simulink library "wheels"  (R2022b)
settings: Solver=VariableStepAuto  StartTime=0.0  StopTime=10.0  RelTol=1e-3
undefined symbols (not defined in the file): raptor_xcp_function
libraries: Raptor_lib x44
settings Model: Creator=serga  LastModifiedBy=serga

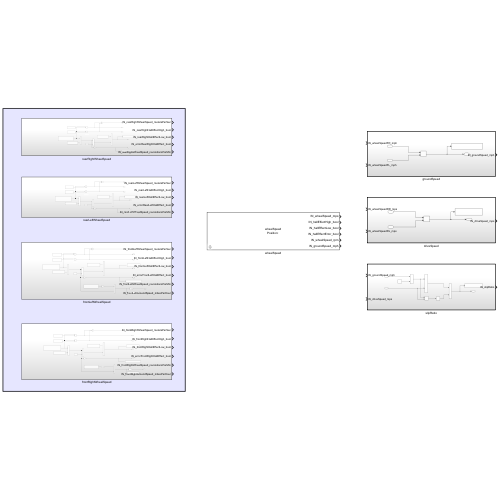
[thumbnail: Simulink's stored preview of the top-level diagram]
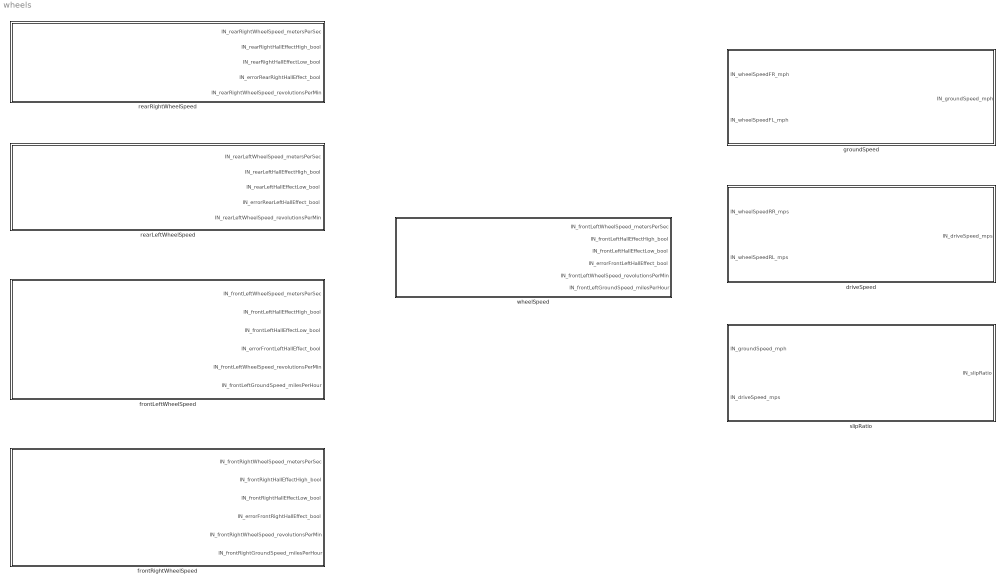
== system wheels ==
  driveSpeed : Subsystem  TreatAsAtomicUnit=on
  frontLeftWheelSpeed : Subsystem
  frontRightWheelSpeed : Subsystem
  groundSpeed : Subsystem  TreatAsAtomicUnit=on
  rearLeftWheelSpeed : Subsystem
  rearRightWheelSpeed : Subsystem
  slipRatio : Subsystem  TreatAsAtomicUnit=on
  wheelSpeed : Subsystem  mask{pos=''}
      mask prompts: pos "Position"
      mask Display:
      | disp(['wheelSpeed\n' ...
      |     'Position: ' pos]);
      | port_label('output', 1, ['IN_wheelSpeed' pos '_mps']);
      | port_label('output', 2, ['IN_hallEffectHigh' pos '_bool']);
      | port_label('output', 3, ['IN_hallEffectLow' pos '_bool']);
      | port_label('output', 4, ['IN_hallEffectError' pos '_bool']);
      | port_label('output', 5, ['IN_wheelSpeed' pos '_rpm']);
      | port_label('output', 6, ['IN_groundSpeed' pos '_mph']);

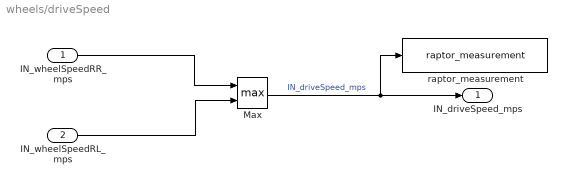
== system wheels/driveSpeed ==
  IN_wheelSpeedRR_mps : Inport
  IN_wheelSpeedRL_mps : Inport  Port=2
  Max : MinMax  Function=max  Inputs=2
  raptor_measurement : Raptor_lib/Data Storage/raptor_measurement  paramName='DataName'  nameSource=Input Wire  calDispType=Number  calEnum={'False', 'True'}  calGain=1.0  calOffset=0.0  calMax=inf  calMin=-inf  calFormat='-1'  calUnit=''  calHelp=''  calAccess=1  calFunction=raptor_xcp_function(gcb)  calVisible=on
      settings: SourceProductName=Raptor
  IN_driveSpeed_mps : Outport
  wires:
  IN_wheelSpeedRL_mps/1 -> Max/2
  Max/1 -> raptor_measurement/1, IN_driveSpeed_mps/1  "IN_driveSpeed_mps"
  IN_wheelSpeedRR_mps/1 -> Max/1

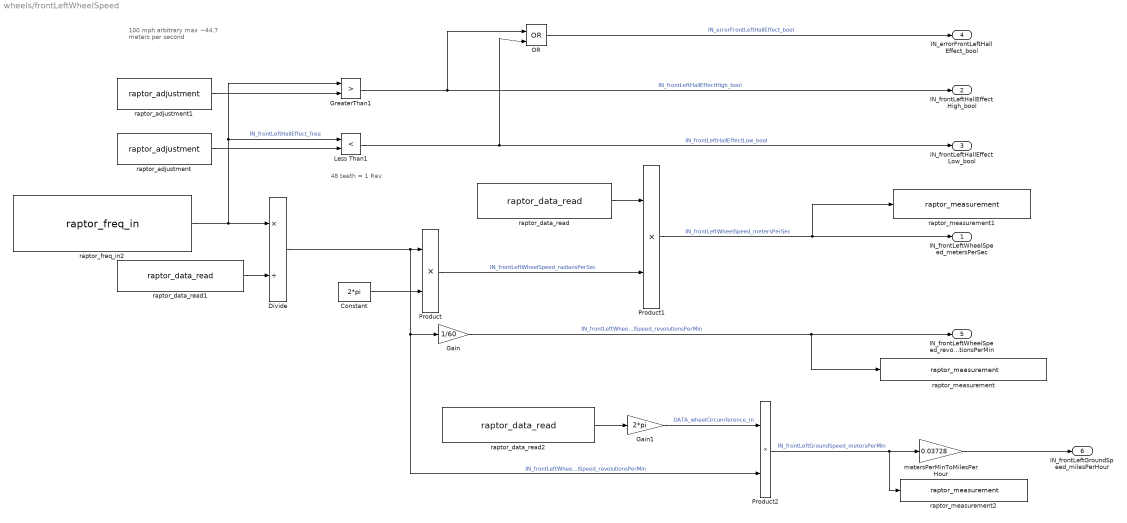
== system wheels/frontLeftWheelSpeed ==
  note: 48 teeth = 1 Rev
  note: 100 mph arbitrary max
      | ~44.7 meters per second
  Constant : Constant  Value=2*pi
  Divide : Product  Inputs=*/
  Gain : Gain  Gain=1/60
  Gain1 : Gain  Gain=2*pi
  GreaterThan1 : RelationalOperator  Operator=>  OutDataTypeStr=boolean  RndMeth=Simplest  InputSameDT=off
  Less Than1 : RelationalOperator  Operator=<  OutDataTypeStr=boolean  RndMeth=Simplest  InputSameDT=off
  OR : Logic  Operator=OR  IconShape=distinctive  AllPortsSameDT=off  OutDataTypeStr=boolean
  Product : Product
  Product1 : Product
  Product2 : Product
  metersPerMinToMilesPerHour : Gain  Gain=0.03728
  raptor_adjustment : Raptor_lib/Data Storage/raptor_adjustment  paramName='IN_frontLeftHallEffectLow_freq'  nameSource=Parameter  initValue=0  dataType=single  storage=Calibration  calDispType=Number  calEnum={'False', 'True'}  calGain=1.0  calOffset=0.0  calMax=inf  calMin=-inf  calFormat='-1'  calUnit=''  calHelp=''  calAccess=1  calFunction=raptor_xcp_function(gcb)  calDispHeaders=off  calColHeaders={'Col1' 'Col2' 'Col3'}  calRowHeaders={'Row1' 'Row2' 'Row3'}
      settings: SourceProductName=Raptor
  raptor_adjustment1 : Raptor_lib/Data Storage/raptor_adjustment  paramName='IN_frontLeftHallEffectHigh_freq'  nameSource=Parameter  initValue=1680  dataType=single  storage=Calibration  calDispType=Number  calEnum={'False', 'True'}  calGain=1.0  calOffset=0.0  calMax=inf  calMin=-inf  calFormat='-1'  calUnit=''  calHelp=''  calAccess=1  calFunction=raptor_xcp_function(gcb)  calDispHeaders=off  calColHeaders={'Col1' 'Col2' 'Col3'}  calRowHeaders={'Row1' 'Row2' 'Row3'}
      settings: SourceProductName=Raptor
  raptor_data_read : Raptor_lib/Data Storage/raptor_data_read  dataName='DATA_unloadedWheelRadius_m'  dataShape=Scalar  idxSource=Input  idxRow=1  idxCol=1
      settings: SourceProductName=Raptor
  raptor_data_read1 : Raptor_lib/Data Storage/raptor_data_read  dataName='DATA_wheelTooth_ct'  dataShape=Scalar  idxSource=Input  idxRow=1  idxCol=1
      settings: SourceProductName=Raptor
  raptor_data_read2 : Raptor_lib/Data Storage/raptor_data_read  dataName='DATA_unloadedWheelRadius_m'  dataShape=Scalar  idxSource=Input  idxRow=1  idxCol=1
      settings: SourceProductName=Raptor
  raptor_freq_in2 : Raptor_lib/Input & Output/raptor_freq_in  resourceValues=INPUT41|INPUT42|INPUT43|INPUT44|INPUT45|(None)  resource=INPUT43  pullUDValues=[]  pullUD=[]  interfaceValues=[]  interface=[]  hasDuty=off  hasEdgeCount='RAPTOR MASK DEFAULT'
      settings: SourceProductName=Raptor
  raptor_measurement : Raptor_lib/Data Storage/raptor_measurement  paramName='DataName'  nameSource=Input Wire  calDispType=Number  calEnum={'False', 'True'}  calGain=1.0  calOffset=0.0  calMax=inf  calMin=-inf  calFormat='-1'  calUnit=''  calHelp=''  calAccess=1  calFunction=raptor_xcp_function(gcb)  calVisible=on
      settings: SourceProductName=Raptor
  raptor_measurement1 : Raptor_lib/Data Storage/raptor_measurement  paramName='DataName'  nameSource=Input Wire  calDispType=Number  calEnum={'False', 'True'}  calGain=1.0  calOffset=0.0  calMax=inf  calMin=-inf  calFormat='-1'  calUnit=''  calHelp=''  calAccess=1  calFunction=raptor_xcp_function(gcb)  calVisible=on
      settings: SourceProductName=Raptor
  raptor_measurement2 : Raptor_lib/Data Storage/raptor_measurement  paramName='DataName'  nameSource=Input Wire  calDispType=Number  calEnum={'False', 'True'}  calGain=1.0  calOffset=0.0  calMax=inf  calMin=-inf  calFormat='-1'  calUnit=''  calHelp=''  calAccess=1  calFunction=raptor_xcp_function(gcb)  calVisible=on
      settings: SourceProductName=Raptor
  IN_frontLeftWheelSpeed_metersPerSec : Outport
  IN_frontLeftHallEffectHigh_bool : Outport  Port=2
  IN_frontLeftHallEffectLow_bool : Outport  Port=3
  IN_errorFrontLeftHallEffect_bool : Outport  Port=4
  IN_frontLeftWheelSpeed_revolutionsPerMin : Outport  Port=5
  IN_frontLeftGroundSpeed_milesPerHour : Outport  Port=6
  wires:
  Product2/1 -> raptor_measurement2/1, metersPerMinToMilesPerHour/1  "IN_frontLeftGroundSpeed_metersPerMin"
  Divide/1 -> Product2/2, Gain/1, Product/1  "IN_frontLeftWheelSpeed_revolutionsPerMin"
  Gain1/1 -> Product2/1  "DATA_wheelCircumference_m"
  raptor_data_read/1 -> Product1/1
  raptor_data_read2/1 -> Gain1/1
  Less Than1/1 -> IN_frontLeftHallEffectLow_bool/1, OR/2  "IN_frontLeftHallEffectLow_bool"
  raptor_freq_in2/1 -> Less Than1/1, GreaterThan1/1, Divide/1  "IN_frontLeftHallEffect_freq"
  metersPerMinToMilesPerHour/1 -> IN_frontLeftGroundSpeed_milesPerHour/1
  Constant/1 -> Product/2
  raptor_adjustment/1 -> Less Than1/2
  OR/1 -> IN_errorFrontLeftHallEffect_bool/1  "IN_errorFrontLeftHallEffect_bool"
  raptor_adjustment1/1 -> GreaterThan1/2
  raptor_data_read1/1 -> Divide/2
  Product1/1 -> raptor_measurement1/1, IN_frontLeftWheelSpeed_metersPerSec/1  "IN_frontLeftWheelSpeed_metersPerSec"
  Gain/1 -> raptor_measurement/1, IN_frontLeftWheelSpeed_revolutionsPerMin/1  "IN_frontLeftWheelSpeed_revolutionsPerMin"
  Product/1 -> Product1/2  "IN_frontLeftWheelSpeed_radiansPerSec"
  GreaterThan1/1 -> IN_frontLeftHallEffectHigh_bool/1, OR/1  "IN_frontLeftHallEffectHigh_bool"

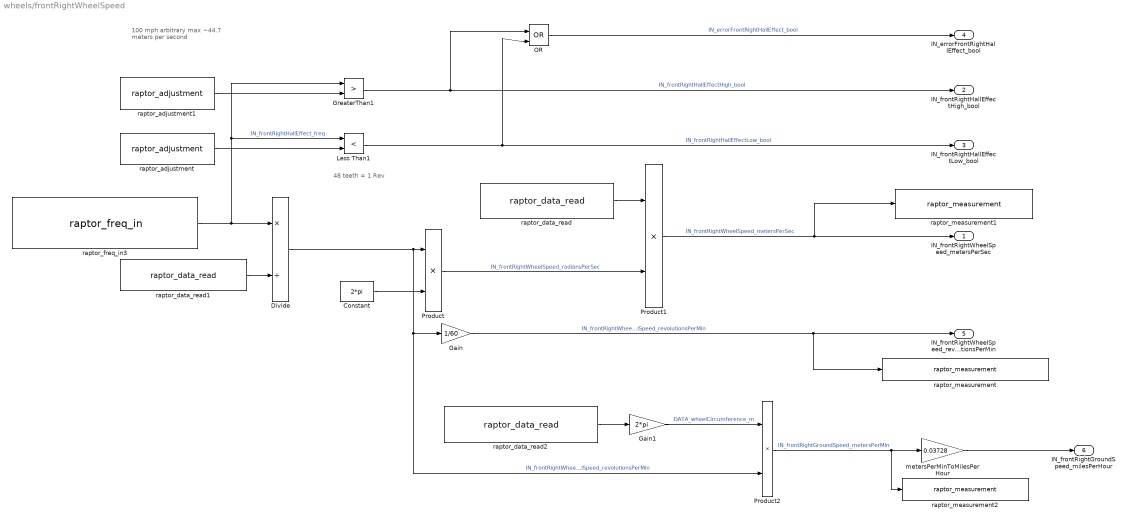
== system wheels/frontRightWheelSpeed ==
  note: 100 mph arbitrary max
      | ~44.7 meters per second
  note: 48 teeth = 1 Rev
  Constant : Constant  Value=2*pi
  Divide : Product  Inputs=*/
  Gain : Gain  Gain=1/60
  Gain1 : Gain  Gain=2*pi
  GreaterThan1 : RelationalOperator  Operator=>  OutDataTypeStr=boolean  RndMeth=Simplest  InputSameDT=off
  Less Than1 : RelationalOperator  Operator=<  OutDataTypeStr=boolean  RndMeth=Simplest  InputSameDT=off
  OR : Logic  Operator=OR  IconShape=distinctive  AllPortsSameDT=off  OutDataTypeStr=boolean
  Product : Product
  Product1 : Product
  Product2 : Product
  metersPerMinToMilesPerHour : Gain  Gain=0.03728
  raptor_adjustment : Raptor_lib/Data Storage/raptor_adjustment  paramName='IN_frontRightHallEffectLow_freq'  nameSource=Parameter  initValue=0  dataType=single  storage=Calibration  calDispType=Number  calEnum={'False', 'True'}  calGain=1.0  calOffset=0.0  calMax=inf  calMin=-inf  calFormat='-1'  calUnit=''  calHelp=''  calAccess=1  calFunction=raptor_xcp_function(gcb)  calDispHeaders=off  calColHeaders={'Col1' 'Col2' 'Col3'}  calRowHeaders={'Row1' 'Row2' 'Row3'}
      settings: SourceProductName=Raptor
  raptor_adjustment1 : Raptor_lib/Data Storage/raptor_adjustment  paramName='IN_frontRightHallEffectHigh_freq'  nameSource=Parameter  initValue=1680  dataType=single  storage=Calibration  calDispType=Number  calEnum={'False', 'True'}  calGain=1.0  calOffset=0.0  calMax=inf  calMin=-inf  calFormat='-1'  calUnit=''  calHelp=''  calAccess=1  calFunction=raptor_xcp_function(gcb)  calDispHeaders=off  calColHeaders={'Col1' 'Col2' 'Col3'}  calRowHeaders={'Row1' 'Row2' 'Row3'}
      settings: SourceProductName=Raptor
  raptor_data_read : Raptor_lib/Data Storage/raptor_data_read  dataName='DATA_unloadedWheelRadius_m'  dataShape=Scalar  idxSource=Input  idxRow=1  idxCol=1
      settings: SourceProductName=Raptor
  raptor_data_read1 : Raptor_lib/Data Storage/raptor_data_read  dataName='DATA_wheelTooth_ct'  dataShape=Scalar  idxSource=Input  idxRow=1  idxCol=1
      settings: SourceProductName=Raptor
  raptor_data_read2 : Raptor_lib/Data Storage/raptor_data_read  dataName='DATA_unloadedWheelRadius_m'  dataShape=Scalar  idxSource=Input  idxRow=1  idxCol=1
      settings: SourceProductName=Raptor
  raptor_freq_in3 : Raptor_lib/Input & Output/raptor_freq_in  resourceValues=INPUT41|INPUT42|INPUT43|INPUT44|INPUT45|(None)  resource=INPUT44  pullUDValues=[]  pullUD=[]  interfaceValues=[]  interface=[]  hasDuty=off  hasEdgeCount='RAPTOR MASK DEFAULT'
      settings: SourceProductName=Raptor
  raptor_measurement : Raptor_lib/Data Storage/raptor_measurement  paramName='DataName'  nameSource=Input Wire  calDispType=Number  calEnum={'False', 'True'}  calGain=1.0  calOffset=0.0  calMax=inf  calMin=-inf  calFormat='-1'  calUnit=''  calHelp=''  calAccess=1  calFunction=raptor_xcp_function(gcb)  calVisible=on
      settings: SourceProductName=Raptor
  raptor_measurement1 : Raptor_lib/Data Storage/raptor_measurement  paramName='DataName'  nameSource=Input Wire  calDispType=Number  calEnum={'False', 'True'}  calGain=1.0  calOffset=0.0  calMax=inf  calMin=-inf  calFormat='-1'  calUnit=''  calHelp=''  calAccess=1  calFunction=raptor_xcp_function(gcb)  calVisible=on
      settings: SourceProductName=Raptor
  raptor_measurement2 : Raptor_lib/Data Storage/raptor_measurement  paramName='DataName'  nameSource=Input Wire  calDispType=Number  calEnum={'False', 'True'}  calGain=1.0  calOffset=0.0  calMax=inf  calMin=-inf  calFormat='-1'  calUnit=''  calHelp=''  calAccess=1  calFunction=raptor_xcp_function(gcb)  calVisible=on
      settings: SourceProductName=Raptor
  IN_frontRightWheelSpeed_metersPerSec : Outport
  IN_frontRightHallEffectHigh_bool : Outport  Port=2
  IN_frontRightHallEffectLow_bool : Outport  Port=3
  IN_errorFrontRightHallEffect_bool : Outport  Port=4
  IN_frontRightWheelSpeed_revolutionsPerMin : Outport  Port=5
  IN_frontRightGroundSpeed_milesPerHour : Outport  Port=6
  wires:
  raptor_adjustment/1 -> Less Than1/2
  raptor_freq_in3/1 -> Less Than1/1, GreaterThan1/1, Divide/1  "IN_frontRightHallEffect_freq"
  raptor_adjustment1/1 -> GreaterThan1/2
  OR/1 -> IN_errorFrontRightHallEffect_bool/1  "IN_errorFrontRightHallEffect_bool"
  GreaterThan1/1 -> IN_frontRightHallEffectHigh_bool/1, OR/1  "IN_frontRightHallEffectHigh_bool"
  Less Than1/1 -> IN_frontRightHallEffectLow_bool/1, OR/2  "IN_frontRightHallEffectLow_bool"
  Gain/1 -> raptor_measurement/1, IN_frontRightWheelSpeed_revolutionsPerMin/1  "IN_frontRightWheelSpeed_revolutionsPerMin"
  raptor_data_read1/1 -> Divide/2
  raptor_data_read/1 -> Product1/1
  Constant/1 -> Product/2
  Product1/1 -> raptor_measurement1/1, IN_frontRightWheelSpeed_metersPerSec/1  "IN_frontRightWheelSpeed_metersPerSec"
  Product/1 -> Product1/2  "IN_frontRightWheelSpeed_radiansPerSec"
  Product2/1 -> raptor_measurement2/1, metersPerMinToMilesPerHour/1  "IN_frontRightGroundSpeed_metersPerMin"
  Gain1/1 -> Product2/1  "DATA_wheelCircumference_m"
  Divide/1 -> Product2/2, Gain/1, Product/1  "IN_frontRightWheelSpeed_revolutionsPerMin"
  raptor_data_read2/1 -> Gain1/1
  metersPerMinToMilesPerHour/1 -> IN_frontRightGroundSpeed_milesPerHour/1

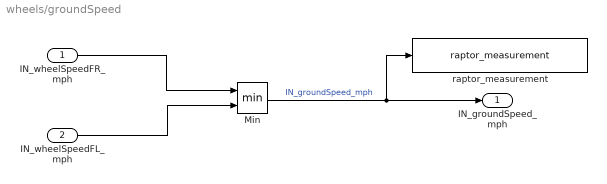
== system wheels/groundSpeed ==
  IN_wheelSpeedFR_mph : Inport
  IN_wheelSpeedFL_mph : Inport  Port=2
  Min : MinMax  Inputs=2
  raptor_measurement : Raptor_lib/Data Storage/raptor_measurement  paramName='DataName'  nameSource=Input Wire  calDispType=Number  calEnum={'False', 'True'}  calGain=1.0  calOffset=0.0  calMax=inf  calMin=-inf  calFormat='-1'  calUnit=''  calHelp=''  calAccess=1  calFunction=raptor_xcp_function(gcb)  calVisible=on
      settings: SourceProductName=Raptor
  IN_groundSpeed_mph : Outport
  wires:
  IN_wheelSpeedFR_mph/1 -> Min/1
  IN_wheelSpeedFL_mph/1 -> Min/2
  Min/1 -> raptor_measurement/1, IN_groundSpeed_mph/1  "IN_groundSpeed_mph"

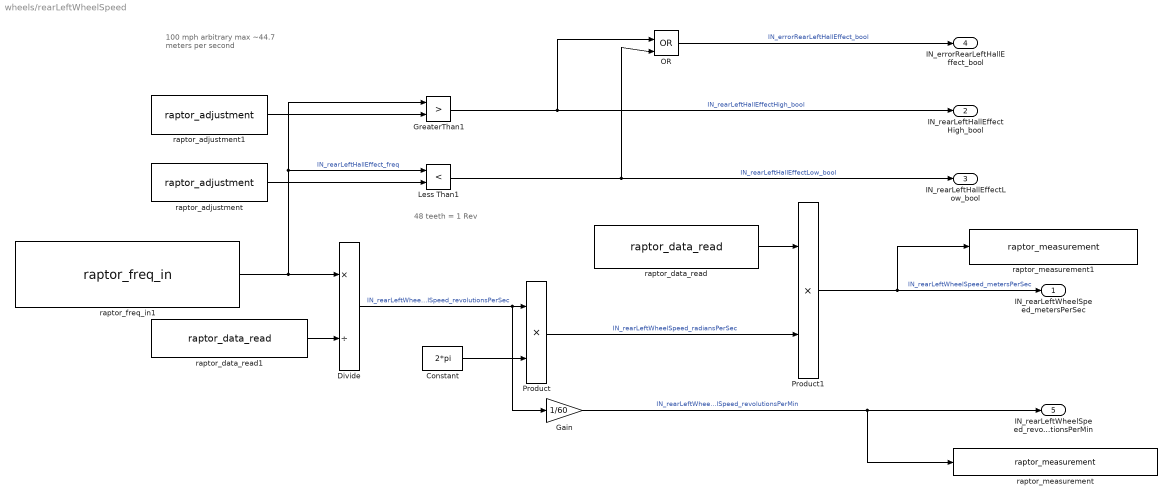
== system wheels/rearLeftWheelSpeed ==
  note: 100 mph arbitrary max
      | ~44.7 meters per second
  note: 48 teeth = 1 Rev
  Constant : Constant  Value=2*pi
  Divide : Product  Inputs=*/
  Gain : Gain  Gain=1/60
  GreaterThan1 : RelationalOperator  Operator=>  OutDataTypeStr=boolean  RndMeth=Simplest  InputSameDT=off
  Less Than1 : RelationalOperator  Operator=<  OutDataTypeStr=boolean  RndMeth=Simplest  InputSameDT=off
  OR : Logic  Operator=OR  IconShape=distinctive  AllPortsSameDT=off  OutDataTypeStr=boolean
  Product : Product
  Product1 : Product
  raptor_adjustment : Raptor_lib/Data Storage/raptor_adjustment  paramName='IN_rearLeftHallEffectLow_freq'  nameSource=Parameter  initValue=0  dataType=single  storage=Calibration  calDispType=Number  calEnum={'False', 'True'}  calGain=1.0  calOffset=0.0  calMax=inf  calMin=-inf  calFormat='-1'  calUnit=''  calHelp=''  calAccess=1  calFunction=raptor_xcp_function(gcb)  calDispHeaders=off  calColHeaders={'Col1' 'Col2' 'Col3'}  calRowHeaders={'Row1' 'Row2' 'Row3'}
      settings: SourceProductName=Raptor
  raptor_adjustment1 : Raptor_lib/Data Storage/raptor_adjustment  paramName='IN_rearLeftHallEffectHigh_freq'  nameSource=Parameter  initValue=1680  dataType=single  storage=Calibration  calDispType=Number  calEnum={'False', 'True'}  calGain=1.0  calOffset=0.0  calMax=inf  calMin=-inf  calFormat='-1'  calUnit=''  calHelp=''  calAccess=1  calFunction=raptor_xcp_function(gcb)  calDispHeaders=off  calColHeaders={'Col1' 'Col2' 'Col3'}  calRowHeaders={'Row1' 'Row2' 'Row3'}
      settings: SourceProductName=Raptor
  raptor_data_read : Raptor_lib/Data Storage/raptor_data_read  dataName='DATA_unloadedWheelRadius_m'  dataShape=Scalar  idxSource=Input  idxRow=1  idxCol=1
      settings: SourceProductName=Raptor
  raptor_data_read1 : Raptor_lib/Data Storage/raptor_data_read  dataName='DATA_wheelTooth_ct'  dataShape=Scalar  idxSource=Input  idxRow=1  idxCol=1
      settings: SourceProductName=Raptor
  raptor_freq_in1 : Raptor_lib/Input & Output/raptor_freq_in  resourceValues=INPUT41|INPUT42|INPUT43|INPUT44|INPUT45|(None)  resource=INPUT42  pullUDValues=[]  pullUD=[]  interfaceValues=[]  interface=[]  hasDuty=off  hasEdgeCount='RAPTOR MASK DEFAULT'
      settings: SourceProductName=Raptor
  raptor_measurement : Raptor_lib/Data Storage/raptor_measurement  paramName='DataName'  nameSource=Input Wire  calDispType=Number  calEnum={'False', 'True'}  calGain=1.0  calOffset=0.0  calMax=inf  calMin=-inf  calFormat='-1'  calUnit=''  calHelp=''  calAccess=1  calFunction=raptor_xcp_function(gcb)  calVisible=on
      settings: SourceProductName=Raptor
  raptor_measurement1 : Raptor_lib/Data Storage/raptor_measurement  paramName='DataName'  nameSource=Input Wire  calDispType=Number  calEnum={'False', 'True'}  calGain=1.0  calOffset=0.0  calMax=inf  calMin=-inf  calFormat='-1'  calUnit=''  calHelp=''  calAccess=1  calFunction=raptor_xcp_function(gcb)  calVisible=on
      settings: SourceProductName=Raptor
  IN_rearLeftWheelSpeed_metersPerSec : Outport
  IN_rearLeftHallEffectHigh_bool : Outport  Port=2
  IN_rearLeftHallEffectLow_bool : Outport  Port=3
  IN_errorRearLeftHallEffect_bool : Outport  Port=4
  IN_rearLeftWheelSpeed_revolutionsPerMin : Outport  Port=5
  wires:
  raptor_adjustment/1 -> Less Than1/2
  raptor_freq_in1/1 -> Less Than1/1, GreaterThan1/1, Divide/1  "IN_rearLeftHallEffect_freq"
  raptor_adjustment1/1 -> GreaterThan1/2
  OR/1 -> IN_errorRearLeftHallEffect_bool/1  "IN_errorRearLeftHallEffect_bool"
  GreaterThan1/1 -> IN_rearLeftHallEffectHigh_bool/1, OR/1  "IN_rearLeftHallEffectHigh_bool"
  Less Than1/1 -> IN_rearLeftHallEffectLow_bool/1, OR/2  "IN_rearLeftHallEffectLow_bool"
  Gain/1 -> IN_rearLeftWheelSpeed_revolutionsPerMin/1, raptor_measurement/1  "IN_rearLeftWheelSpeed_revolutionsPerMin"
  raptor_data_read1/1 -> Divide/2
  raptor_data_read/1 -> Product1/1
  Divide/1 -> Gain/1, Product/1  "IN_rearLeftWheelSpeed_revolutionsPerSec"
  Constant/1 -> Product/2
  Product1/1 -> raptor_measurement1/1, IN_rearLeftWheelSpeed_metersPerSec/1  "IN_rearLeftWheelSpeed_metersPerSec"
  Product/1 -> Product1/2  "IN_rearLeftWheelSpeed_radiansPerSec"

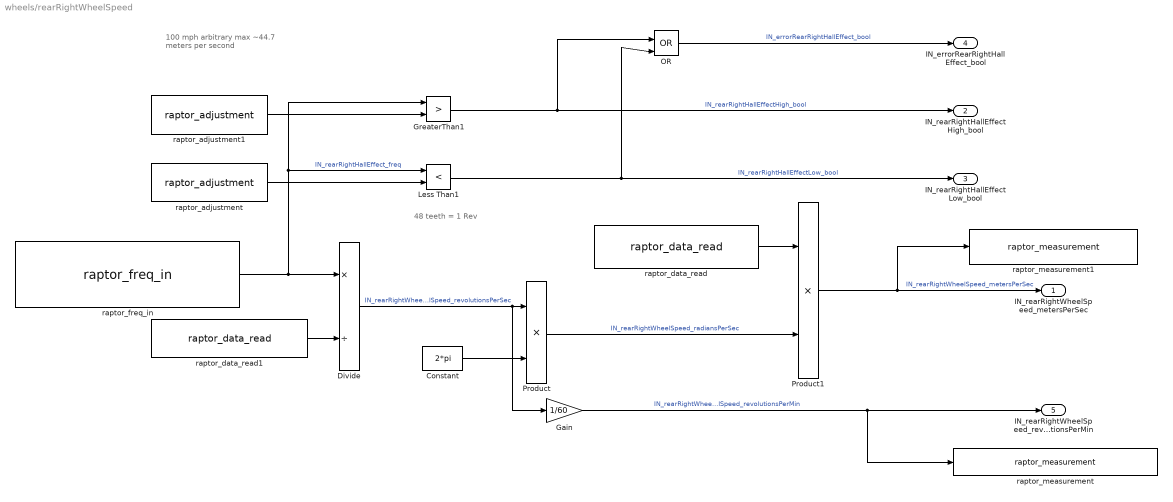
== system wheels/rearRightWheelSpeed ==
  note: 100 mph arbitrary max
      | ~44.7 meters per second
  note: 48 teeth = 1 Rev
  Constant : Constant  Value=2*pi
  Divide : Product  Inputs=*/
  Gain : Gain  Gain=1/60
  GreaterThan1 : RelationalOperator  Operator=>  OutDataTypeStr=boolean  RndMeth=Simplest  InputSameDT=off
  Less Than1 : RelationalOperator  Operator=<  OutDataTypeStr=boolean  RndMeth=Simplest  InputSameDT=off
  OR : Logic  Operator=OR  IconShape=distinctive  AllPortsSameDT=off  OutDataTypeStr=boolean
  Product : Product
  Product1 : Product
  raptor_adjustment : Raptor_lib/Data Storage/raptor_adjustment  paramName='IN_rearRightHallEffectLow_freq'  nameSource=Parameter  initValue=0  dataType=single  storage=Calibration  calDispType=Number  calEnum={'False', 'True'}  calGain=1.0  calOffset=0.0  calMax=inf  calMin=-inf  calFormat='-1'  calUnit=''  calHelp=''  calAccess=1  calFunction=raptor_xcp_function(gcb)  calDispHeaders=off  calColHeaders={'Col1' 'Col2' 'Col3'}  calRowHeaders={'Row1' 'Row2' 'Row3'}
      settings: SourceProductName=Raptor
  raptor_adjustment1 : Raptor_lib/Data Storage/raptor_adjustment  paramName='IN_rearRightHallEffectHigh_freq'  nameSource=Parameter  initValue=1680  dataType=single  storage=Calibration  calDispType=Number  calEnum={'False', 'True'}  calGain=1.0  calOffset=0.0  calMax=inf  calMin=-inf  calFormat='-1'  calUnit=''  calHelp=''  calAccess=1  calFunction=raptor_xcp_function(gcb)  calDispHeaders=off  calColHeaders={'Col1' 'Col2' 'Col3'}  calRowHeaders={'Row1' 'Row2' 'Row3'}
      settings: SourceProductName=Raptor
  raptor_data_read : Raptor_lib/Data Storage/raptor_data_read  dataName='DATA_unloadedWheelRadius_m'  dataShape=Scalar  idxSource=Input  idxRow=1  idxCol=1
      settings: SourceProductName=Raptor
  raptor_data_read1 : Raptor_lib/Data Storage/raptor_data_read  dataName='DATA_wheelTooth_ct'  dataShape=Scalar  idxSource=Input  idxRow=1  idxCol=1
      settings: SourceProductName=Raptor
  raptor_freq_in : Raptor_lib/Input & Output/raptor_freq_in  resourceValues=INPUT41|INPUT42|INPUT43|INPUT44|INPUT45|(None)  resource=INPUT41  pullUDValues=[]  pullUD=[]  interfaceValues=[]  interface=[]  hasDuty=off  hasEdgeCount='RAPTOR MASK DEFAULT'
      settings: SourceProductName=Raptor
  raptor_measurement : Raptor_lib/Data Storage/raptor_measurement  paramName='DataName'  nameSource=Input Wire  calDispType=Number  calEnum={'False', 'True'}  calGain=1.0  calOffset=0.0  calMax=inf  calMin=-inf  calFormat='-1'  calUnit=''  calHelp=''  calAccess=1  calFunction=raptor_xcp_function(gcb)  calVisible=on
      settings: SourceProductName=Raptor
  raptor_measurement1 : Raptor_lib/Data Storage/raptor_measurement  paramName='DataName'  nameSource=Input Wire  calDispType=Number  calEnum={'False', 'True'}  calGain=1.0  calOffset=0.0  calMax=inf  calMin=-inf  calFormat='-1'  calUnit=''  calHelp=''  calAccess=1  calFunction=raptor_xcp_function(gcb)  calVisible=on
      settings: SourceProductName=Raptor
  IN_rearRightWheelSpeed_metersPerSec : Outport
  IN_rearRightHallEffectHigh_bool : Outport  Port=2
  IN_rearRightHallEffectLow_bool : Outport  Port=3
  IN_errorRearRightHallEffect_bool : Outport  Port=4
  IN_rearRightWheelSpeed_revolutionsPerMin : Outport  Port=5
  wires:
  raptor_data_read1/1 -> Divide/2
  Divide/1 -> Gain/1, Product/1  "IN_rearRightWheelSpeed_revolutionsPerSec"
  Constant/1 -> Product/2
  Product/1 -> Product1/2  "IN_rearRightWheelSpeed_radiansPerSec"
  raptor_data_read/1 -> Product1/1
  Product1/1 -> raptor_measurement1/1, IN_rearRightWheelSpeed_metersPerSec/1  "IN_rearRightWheelSpeed_metersPerSec"
  raptor_freq_in/1 -> Less Than1/1, GreaterThan1/1, Divide/1  "IN_rearRightHallEffect_freq"
  raptor_adjustment1/1 -> GreaterThan1/2
  raptor_adjustment/1 -> Less Than1/2
  Less Than1/1 -> IN_rearRightHallEffectLow_bool/1, OR/2  "IN_rearRightHallEffectLow_bool"
  OR/1 -> IN_errorRearRightHallEffect_bool/1  "IN_errorRearRightHallEffect_bool"
  GreaterThan1/1 -> IN_rearRightHallEffectHigh_bool/1, OR/1  "IN_rearRightHallEffectHigh_bool"
  Gain/1 -> IN_rearRightWheelSpeed_revolutionsPerMin/1, raptor_measurement/1  "IN_rearRightWheelSpeed_revolutionsPerMin"

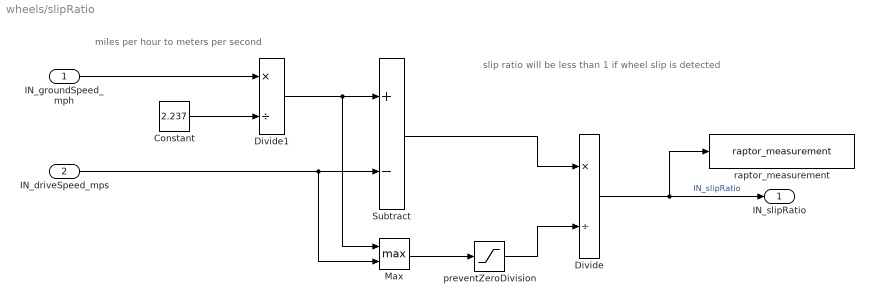
== system wheels/slipRatio ==
  note: slip ratio will be less than 1 if wheel slip is detected
  note: miles per hour to meters per second
  IN_groundSpeed_mph : Inport
  IN_driveSpeed_mps : Inport  Port=2
  Constant : Constant  Value=2.237
  Divide : Product  Inputs=*/
  Divide1 : Product  Inputs=*/
  Max : MinMax  Function=max  Inputs=2
  Subtract : Sum  Inputs=+-
  preventZeroDivision : Saturate  UpperLimit=1000  LowerLimit=0.0001
  raptor_measurement : Raptor_lib/Data Storage/raptor_measurement  paramName='DataName'  nameSource=Input Wire  calDispType=Number  calEnum={'False', 'True'}  calGain=1.0  calOffset=0.0  calMax=inf  calMin=-inf  calFormat='-1'  calUnit=''  calHelp=''  calAccess=1  calFunction=raptor_xcp_function(gcb)  calVisible=on
      settings: SourceProductName=Raptor
  IN_slipRatio : Outport
  wires:
  Divide/1 -> raptor_measurement/1, IN_slipRatio/1  "IN_slipRatio"
  IN_groundSpeed_mph/1 -> Divide1/1
  Constant/1 -> Divide1/2
  IN_driveSpeed_mps/1 -> Max/2, Subtract/2
  Divide1/1 -> Max/1, Subtract/1
  Subtract/1 -> Divide/1
  Max/1 -> preventZeroDivision/1
  preventZeroDivision/1 -> Divide/2

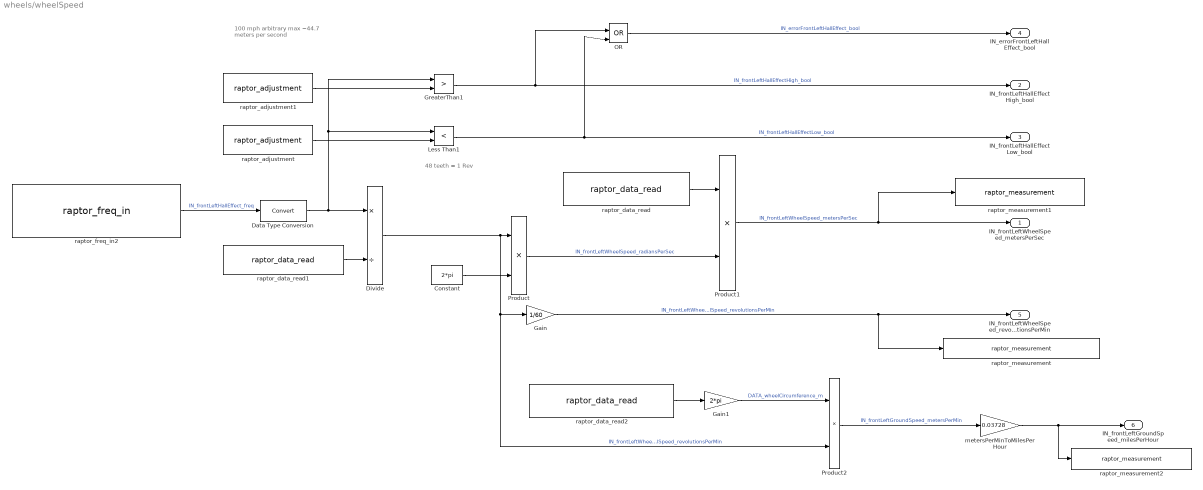
== system wheels/wheelSpeed ==
  note: 48 teeth = 1 Rev
  note: 100 mph arbitrary max
      | ~44.7 meters per second
  Constant : Constant  Value=2*pi
  Data Type Conversion : DataTypeConversion  SaturateOnIntegerOverflow=off  RndMeth=Floor
  Divide : Product  Inputs=*/
  Gain : Gain  Gain=1/60
  Gain1 : Gain  Gain=2*pi
  GreaterThan1 : RelationalOperator  Operator=>  OutDataTypeStr=boolean  RndMeth=Simplest  InputSameDT=off
  Less Than1 : RelationalOperator  Operator=<  OutDataTypeStr=boolean  RndMeth=Simplest  InputSameDT=off
  OR : Logic  Operator=OR  IconShape=distinctive  AllPortsSameDT=off  OutDataTypeStr=boolean
  Product : Product
  Product1 : Product
  Product2 : Product
  metersPerMinToMilesPerHour : Gain  Gain=0.03728
  raptor_adjustment : Raptor_lib/Data Storage/raptor_adjustment  paramName=['IN_hallEffectLow' pos '_hz']  nameSource=Parameter  initValue=0  dataType=single  storage=Calibration  calDispType=Number  calEnum={'False', 'True'}  calGain=1.0  calOffset=0.0  calMax=inf  calMin=-inf  calFormat='-1'  calUnit=''  calHelp=''  calAccess=1  calFunction=raptor_xcp_function(gcb)  calDispHeaders=off  calColHeaders={'Col1' 'Col2' 'Col3'}  calRowHeaders={'Row1' 'Row2' 'Row3'}
      settings: SourceProductName=Raptor
  raptor_adjustment1 : Raptor_lib/Data Storage/raptor_adjustment  paramName=['IN_hallEffectHigh' pos '_hz']  nameSource=Parameter  initValue=1680  dataType=single  storage=Calibration  calDispType=Number  calEnum={'False', 'True'}  calGain=1.0  calOffset=0.0  calMax=inf  calMin=-inf  calFormat='-1'  calUnit=''  calHelp=''  calAccess=1  calFunction=raptor_xcp_function(gcb)  calDispHeaders=off  calColHeaders={'Col1' 'Col2' 'Col3'}  calRowHeaders={'Row1' 'Row2' 'Row3'}
      settings: SourceProductName=Raptor
  raptor_data_read : Raptor_lib/Data Storage/raptor_data_read  dataName='DATA_unloadedWheelRadius_m'  dataShape=Scalar  idxSource=Input  idxRow=1  idxCol=1
      settings: SourceProductName=Raptor
  raptor_data_read1 : Raptor_lib/Data Storage/raptor_data_read  dataName='DATA_wheelTooth_ct'  dataShape=Scalar  idxSource=Input  idxRow=1  idxCol=1
      settings: SourceProductName=Raptor
  raptor_data_read2 : Raptor_lib/Data Storage/raptor_data_read  dataName='DATA_unloadedWheelRadius_m'  dataShape=Scalar  idxSource=Input  idxRow=1  idxCol=1
      settings: SourceProductName=Raptor
  raptor_freq_in2 : Raptor_lib/Input & Output/raptor_freq_in  resourceValues=INPUT41|INPUT42|INPUT43|INPUT44|INPUT45|(None)  resource=INPUT43  pullUDValues=[]  pullUD=[]  interfaceValues=[]  interface=[]  hasDuty=off  hasEdgeCount='RAPTOR MASK DEFAULT'
      settings: SourceProductName=Raptor
  raptor_measurement : Raptor_lib/Data Storage/raptor_measurement  paramName=['IN_wheelSpeed' pos '_rpm']  nameSource=Parameter  calDispType=Number  calEnum={'False', 'True'}  calGain=1.0  calOffset=0.0  calMax=inf  calMin=-inf  calFormat='-1'  calUnit=''  calHelp=''  calAccess=1  calFunction=raptor_xcp_function(gcb)  calVisible=on
      settings: SourceProductName=Raptor
  raptor_measurement1 : Raptor_lib/Data Storage/raptor_measurement  paramName=['IN_wheelSpeed' pos '_mps']  nameSource=Parameter  calDispType=Number  calEnum={'False', 'True'}  calGain=1.0  calOffset=0.0  calMax=inf  calMin=-inf  calFormat='-1'  calUnit=''  calHelp=''  calAccess=1  calFunction=raptor_xcp_function(gcb)  calVisible=on
      settings: SourceProductName=Raptor
  raptor_measurement2 : Raptor_lib/Data Storage/raptor_measurement  paramName=['IN_groundSpeed' pos '_mph']  nameSource=Parameter  calDispType=Number  calEnum={'False', 'True'}  calGain=1.0  calOffset=0.0  calMax=inf  calMin=-inf  calFormat='-1'  calUnit=''  calHelp=''  calAccess=1  calFunction=raptor_xcp_function(gcb)  calVisible=on
      settings: SourceProductName=Raptor
  IN_frontLeftWheelSpeed_metersPerSec : Outport
  IN_frontLeftHallEffectHigh_bool : Outport  Port=2
  IN_frontLeftHallEffectLow_bool : Outport  Port=3
  IN_errorFrontLeftHallEffect_bool : Outport  Port=4
  IN_frontLeftWheelSpeed_revolutionsPerMin : Outport  Port=5
  IN_frontLeftGroundSpeed_milesPerHour : Outport  Port=6
  wires:
  raptor_data_read1/1 -> Divide/2
  metersPerMinToMilesPerHour/1 -> raptor_measurement2/1, IN_frontLeftGroundSpeed_milesPerHour/1
  OR/1 -> IN_errorFrontLeftHallEffect_bool/1  "IN_errorFrontLeftHallEffect_bool"
  raptor_data_read2/1 -> Gain1/1
  Constant/1 -> Product/2
  raptor_freq_in2/1 -> Data Type Conversion/1  "IN_frontLeftHallEffect_freq"
  Less Than1/1 -> IN_frontLeftHallEffectLow_bool/1, OR/2  "IN_frontLeftHallEffectLow_bool"
  Product2/1 -> metersPerMinToMilesPerHour/1  "IN_frontLeftGroundSpeed_metersPerMin"
  raptor_adjustment/1 -> Less Than1/2
  Gain1/1 -> Product2/1  "DATA_wheelCircumference_m"
  GreaterThan1/1 -> IN_frontLeftHallEffectHigh_bool/1, OR/1  "IN_frontLeftHallEffectHigh_bool"
  Product/1 -> Product1/2  "IN_frontLeftWheelSpeed_radiansPerSec"
  Divide/1 -> Product2/2, Gain/1, Product/1  "IN_frontLeftWheelSpeed_revolutionsPerMin"
  raptor_data_read/1 -> Product1/1
  Gain/1 -> raptor_measurement/1, IN_frontLeftWheelSpeed_revolutionsPerMin/1  "IN_frontLeftWheelSpeed_revolutionsPerMin"
  Product1/1 -> raptor_measurement1/1, IN_frontLeftWheelSpeed_metersPerSec/1  "IN_frontLeftWheelSpeed_metersPerSec"
  raptor_adjustment1/1 -> GreaterThan1/2
  Data Type Conversion/1 -> Less Than1/1, GreaterThan1/1, Divide/1
